simulink model "VCU_SW_1"  (R2023b)
settings: Solver=FixedStepDiscrete  StartTime=0.0  StopTime=inf  FixedStep=1e-2  RelTol=1e-3
PreLoadFcn:
  | RTWConfigurationCB('preloadfcn', bdroot);
InitFcn:
  | loadvar_ttc500
undefined symbols (not defined in the file): BrkPedalTypes, CabMovModeTypes, cFuseTempSensAcc_X, cFuseTempSensAcc_Y, cFuseTempSensVal_X, cFuseTempSensVal_Y, cTMSTempSensVal_X, cTMSTempSensVal_Y, cTransferCaseSpeedRatio, diag_state, DoorsPositionTypes, dP_filter_Y, DriverOccClassSystemTypes, ErrorValueTypes, fatal_error_callback, IO_ADC_NO_RANGE, LadderStatusTypes, pAnalogCabRotSensAcc, pAnalogCabRotSensMaxVolt, pAnalogCabRotSensMinVolt, pAnalogCabRotSensRange, pAnalogCabRotSensZeroVolt, pBrkActivePress, pCabTiltSensAcc, pCabTiltSensMaxCur, pCabTiltSensMinCur, pDistanceCorrection, pECANManual_BPNEnable, pECANManual_BPNEnabler_Flag, pFilterSensAccRes, pHDirMaxDiffFrq, pHDirSensHighLvl, pHDirSensLowLvl, pMainGearRatio, pMaxFilterSensRes, pMaxFirstPedalSensValue, pMaxFuseTempSensRes, pMaxPressLoss, pMaxPressSensCurrent, pMaxPressValue, pMaxPressValueHydMotAndPump, pMaxPressValueParkDrain, pMaxSecondPedalSensValue, pMaxTempSensVoltage, pMaxTempValue, pMaxTMSTempSensRes, pMinFilterSensRes, pMinFirstPedalSensValue, pMinFuseTempSensRes, pMinPressLoss, pMinPressSensCurrent, pMinPressValue, pMinSecondPedalSensValue, pMinTempSensVoltage, pMinTempValue, pMinTMSTempSensRes, pMotorRingTeethNum, pPedalSensAccuracyPct, pPedalSensAccuracyVolt, pPressLossTreshhold ... (+20)
libraries: TTlibrary x270, canmsglib x127, simulink x88
(part 2 of 19)

== system VCU_SW_1/ServerFcn/convDiagDataForTest ==
  convDiagDataForTest : TriggerPort  TriggerType=function-call  IsSimulinkFunction=on  FunctionName=convDiagDataForTest  VariantControl=(inherit)
  MATLAB Function : MATLAB Function  TreatAsAtomicUnit=on
  rawValue : ArgIn  DisableCoverage=on  OutDataTypeStr=uint16  ArgumentName=rawValue
  finalValue : ArgOut  DisableCoverage=on  OutDataTypeStr=uint8  ArgumentName=finalValue
  wires:
  MATLAB Function/1(canDiag) -> finalValue/1
  rawValue/1 -> MATLAB Function/1(hwDiag)

== system VCU_SW_1/ServerFcn/convINint1 ==
  convINint16fromUint16 : TriggerPort  TriggerType=function-call  IsSimulinkFunction=on  FunctionName=convINint16fromUint16  VariantControl=(inherit)
  MATLAB Function2 : MATLAB Function  TreatAsAtomicUnit=on
  x : ArgIn  DisableCoverage=on  OutDataTypeStr=int16  ArgumentName=x
  y : ArgOut  DisableCoverage=on  OutDataTypeStr=int16  ArgumentName=y
  wires:
  MATLAB Function2/1(y) -> y/1
  x/1 -> MATLAB Function2/1(x)

== system VCU_SW_1/ServerFcn/convINint16 ==
  convINint16 : TriggerPort  TriggerType=function-call  IsSimulinkFunction=on  FunctionName=convINint16  VariantControl=(inherit)
  MATLAB Function2 : MATLAB Function  TreatAsAtomicUnit=on
  x : ArgIn  DisableCoverage=on  OutDataTypeStr=single  ArgumentName=x
  y : ArgOut  DisableCoverage=on  OutDataTypeStr=int16  ArgumentName=y
  wires:
  MATLAB Function2/1(y) -> y/1
  x/1 -> MATLAB Function2/1(x)

== system VCU_SW_1/ServerFcn/convINuint16 ==
  convINuint16 : TriggerPort  TriggerType=function-call  IsSimulinkFunction=on  FunctionName=convINuint16  VariantControl=(inherit)
  MATLAB Function2 : MATLAB Function  TreatAsAtomicUnit=on
  x : ArgIn  DisableCoverage=on  OutDataTypeStr=single  ArgumentName=x
  y : ArgOut  DisableCoverage=on  OutDataTypeStr=uint16  ArgumentName=y
  wires:
  MATLAB Function2/1(y) -> y/1
  x/1 -> MATLAB Function2/1(x)

== system VCU_SW_1/ServerFcn/convPWDData ==
  convPWDData : TriggerPort  TriggerType=function-call  IsSimulinkFunction=on  FunctionName=convPWDData  VariantControl=(inherit)
  MATLAB Function : MATLAB Function  TreatAsAtomicUnit=on
  rawValue : ArgIn  DisableCoverage=on  OutDataTypeStr=uint32  ArgumentName=rawValue
  errorSts : ArgIn  Port=2  OutDataTypeStr=uint16  ArgumentName=errorSts
  finalValue : ArgOut  DisableCoverage=on  OutDataTypeStr=uint16  ArgumentName=finalValue
  wires:
  errorSts/1 -> MATLAB Function/2(errorSts)
  rawValue/1 -> MATLAB Function/1(inpValue)
  MATLAB Function/1(outValue) -> finalValue/1

== system VCU_SW_1/ServerFcn/convPWDDiagDataToEnum ==
  convPWDDiagDataToEnum : TriggerPort  TriggerType=function-call  IsSimulinkFunction=on  FunctionName=convPWDDiagDataToEnum  VariantControl=(inherit)
  Ground : Ground
  Terminator : Terminator
  rawValue : ArgIn  DisableCoverage=on  OutDataTypeStr=uint16  ArgumentName=rawValue
  enumValue : ArgOut  DisableCoverage=on  OutDataTypeStr=Enum: DigitalPinStatusTypes  ArgumentName=enumValue
  wires:
  Ground/1 -> enumValue/1
  rawValue/1 -> Terminator/1

== system VCU_SW_1/ServerFcn/convPWMDiagDataToEnum ==
  convPWMDiagDataToEnum : TriggerPort  TriggerType=function-call  IsSimulinkFunction=on  FunctionName=convPWMDiagDataToEnum  VariantControl=(inherit)
  Ground : Ground
  Terminator : Terminator
  rawValue : ArgIn  DisableCoverage=on  OutDataTypeStr=uint16  ArgumentName=rawValue
  enumValue : ArgOut  DisableCoverage=on  OutDataTypeStr=Enum: DigitalPinStatusTypes  ArgumentName=enumValue
  wires:
  Ground/1 -> enumValue/1
  rawValue/1 -> Terminator/1

== system VCU_SW_1/ServerFcn/convUintPinToenumStt ==
  convUintPinToenumStt : TriggerPort  TriggerType=function-call  IsSimulinkFunction=on  FunctionName=convUintPinToenumStt  VariantControl=(inherit)
  MATLAB Function : MATLAB Function  TreatAsAtomicUnit=on
  uintValue : ArgIn  DisableCoverage=on  OutDataTypeStr=uint8  ArgumentName=uintValue
  rawValue : ArgOut  DisableCoverage=on  OutDataTypeStr=Enum: StateModeTypes  ArgumentName=rawValue
  wires:
  uintValue/1 -> MATLAB Function/1(uintValue)
  MATLAB Function/1(enum) -> rawValue/1

== system VCU_SW_1/logSignal/getDAQCmd ==
  getDAQCmd : TriggerPort  TriggerType=function-call  IsSimulinkFunction=on  FunctionName=getDAQCmd  FunctionVisibility=scoped  VariantControl=(inherit)
  Constant : Constant  Value=uint8(1)
  Constant1 : Constant  Value=uint8(0)
  Constant2 : Constant  Value=uint8(0)
  Constant3 : Constant  Value=uint8(3)
  Terminator{,1..4} (5 alike) : Terminator
  daq_cmd_unpack : canmsglib/CAN Unpack  MsgList=(none)  MsgName=DAQ_CMD  MsgIDType=Extended (29-bit identifier)  MsgIdentifier=419364344  MsgLength=8  SignalInfo={ 'daq_cmd_ena', '0', '8', 'LE', 'unsigned', 'Standard', '0', '1', '0', '0', '255'; 'daq_cmd_page_list', '24', '8', 'LE', 'unsigned', 'Standard', '0', '1', '0', '0', '255'; 'daq_cmd_page_mode', '8', '8', 'LE', 'unsigned', 'Standard', '0', '1', '0', '0', '255'; 'daq_cmd_page_num', '16', '8', 'LE', 'unsigned', 'Standard', '0', '1', '0', '0', '255' }  IDPort=off  TimestampPort=off  ErrorPort=off  RemotePort=off  LengthPort=off  StatusPort=off  ApplyMinMax=off
  read_daq_cmd_msg : TTlibrary/CAN/read_message_name  channel=IO_CAN_CHANNEL_6  id_format=IO_CAN_EXT_FRAME  get_msg_info=off  message_names=there is no CAN Unpack blocks  message_info=|  id=419364344  ac_mask=536870911  retranslation=off  io_error=on  sample_time=-1
      | Message Name: DAQ_CMD
      |  Message ID Type: Standard (11-bit identifier)
      |  Message ID: 2
      settings: SourceProductName=TT control 500 series
  daqEna : ArgOut  OutDataTypeStr=uint8  ArgumentName=daqEna
  daqPage : ArgOut  Port=2  OutDataTypeStr=uint8  ArgumentName=daqPage
  daqList : ArgOut  Port=3  OutDataTypeStr=uint8  ArgumentName=daqList
  daqMode : ArgOut  Port=4  OutDataTypeStr=uint8  ArgumentName=daqMode
  wires:
  read_daq_cmd_msg/2 -> Terminator/1  "handler_err_419364344"
  read_daq_cmd_msg/1 -> daq_cmd_unpack/1  "msg_419364344"
  daq_cmd_unpack/1 -> Terminator1/1
  daq_cmd_unpack/2 -> Terminator2/1
  daq_cmd_unpack/3 -> Terminator3/1
  daq_cmd_unpack/4 -> Terminator4/1
  Constant/1 -> daqEna/1
  Constant1/1 -> daqMode/1
  Constant2/1 -> daqList/1
  Constant3/1 -> daqPage/1

== system VCU_SW_1/logSignal/getListData ==
  getListData : TriggerPort  TriggerType=function-call  IsSimulinkFunction=on  FunctionName=getListData  FunctionVisibility=scoped  VariantControl=(inherit)
  Simulink Function : Subsystem  TreatAsAtomicUnit=on
  Simulink Function1 : Subsystem  TreatAsAtomicUnit=on
  listData_mf : MATLAB Function  TreatAsAtomicUnit=on
  pageHighvoltageAppData : Subsystem  TreatAsAtomicUnit=on
  pageInputFcns : Subsystem  Commented=on  TreatAsAtomicUnit=on
  pageOutputRawData : Subsystem  TreatAsAtomicUnit=on
  pageRawInput : Subsystem  TreatAsAtomicUnit=on
  page : ArgIn  DisableCoverage=on  OutDataTypeStr=uint8  ArgumentName=page
  list : ArgIn  Port=2  OutDataTypeStr=uint8  ArgumentName=list
  data : ArgOut  DisableCoverage=on  OutDataTypeStr=uint8  PortDimensions=[1,7]  ArgumentName=data
  len : ArgOut  Port=2  OutDataTypeStr=uint8  ArgumentName=len
  wires:
  listData_mf/1(data) -> data/1
  listData_mf/2(len) -> len/1
  page/1 -> listData_mf/1(page)
  list/1 -> listData_mf/2(list)

== system VCU_SW_1/logSignal/getListNum ==
  getListNum : TriggerPort  TriggerType=function-call  IsSimulinkFunction=on  FunctionName=getListNum  FunctionVisibility=scoped  VariantControl=(inherit)
  MATLAB Function : MATLAB Function  TreatAsAtomicUnit=on
  page : ArgIn  DisableCoverage=on  OutDataTypeStr=uint8  ArgumentName=page
  num : ArgOut  DisableCoverage=on  OutDataTypeStr=uint8  ArgumentName=num
  wires:
  page/1 -> MATLAB Function/1(pageNum)
  MATLAB Function/1(numList) -> num/1

== system VCU_SW_1/logSignal/transmitDAQMsg ==
  transmitDAQMsg : TriggerPort  TriggerType=function-call  IsSimulinkFunction=on  FunctionName=transmitDAQMsg  FunctionVisibility=scoped  VariantControl=(inherit)
  daqPack : canmsglib/CAN Pack  MsgList=(none)  MsgName=daqPack  MsgIDType=Extended (29-bit identifier)  MsgIdentifier=419364606  MsgLength=8  Remote=off  ApplyMinMax=off  BusOutput=on  SignalInfo={}
      settings: DataFormat=raw data
  transmit_daq : TTlibrary/CAN/transmit_message_name  channel=IO_CAN_CHANNEL_6  id_format=IO_CAN_EXT_FRAME  retranslation=off  io_error=off  sample_time=-1
      settings: SourceProductName=TT control 500 series
  buffer : ArgIn  DisableCoverage=on  OutDataTypeStr=uint8  PortDimensions=[1,8]  ArgumentName=buffer
  wires:
  buffer/1 -> daqPack/1
  daqPack/1 -> transmit_daq/1

== system VCU_SW_1/EEPROM Layer/calculate trip distance/EEPROM read ==
  In1 : Inport
  function : TriggerPort  TriggerType=function-call  VariantControl=Variant
  Data Store Read1 : DataStoreRead  DataStoreName=EEPROMData  DataStoreElements=EEPROMData.savedDistM#EEPROMData.savedDistKM#EEPROMData.savedDistKKM  IndexOptions=Index vector (dialog)  Indices=1  OutputSizes=1
  Data Store Write1 : DataStoreWrite  DataStoreName=EEPROMData  DataStoreElements=EEPROMData.updatedDistM#EEPROMData.updatedDistKM#EEPROMData.updatedDistKKM  IndexOptions=Index vector (dialog)  Indices=1  OutputSizes=1
  Data Store Write2 : DataStoreWrite  DataStoreName=EEPROMData  DataStoreElements=EEPROMData.totalDistM  IndexOptions=Index vector (dialog)  Indices=1  OutputSizes=1
  Display : Display
  calcTotalDist : MATLAB Function  TreatAsAtomicUnit=on
  wires:
  calcTotalDist/4(updDistTotal) -> Display/1, Data Store Write2/1
  calcTotalDist/2(updDistKM) -> Data Store Write1/2
  Data Store Read1/1 -> calcTotalDist/2(savedDistM)
  calcTotalDist/1(updDistM) -> Data Store Write1/1
  In1/1 -> calcTotalDist/1(tripDist)
  Data Store Read1/2 -> calcTotalDist/3(savedDistKM)
  Data Store Read1/3 -> calcTotalDist/4(savedDistKKM)
  calcTotalDist/3(updDistKKM) -> Data Store Write1/3

== system VCU_SW_1/EEPROM Layer/calculate trip distance/EEPROM read1 ==
  In1 : Inport
  function : TriggerPort  TriggerType=function-call  VariantControl=Variant
  Data Store Read1 : DataStoreRead  DataStoreName=EEPROMData  DataStoreElements=EEPROMData.savedDistM_Trip#EEPROMData.savedDistKM_Trip#EEPROMData.savedDistKKM_Trip  IndexOptions=Index vector (dialog)  Indices=1  OutputSizes=1
  Data Store Write1 : DataStoreWrite  DataStoreName=EEPROMData  DataStoreElements=EEPROMData.updatedDistM_Trip#EEPROMData.updatedDistKM_Trip#EEPROMData.updatedDistKKM_Trip  IndexOptions=Index vector (dialog)  Indices=1  OutputSizes=1
  Data Store Write2 : DataStoreWrite  DataStoreName=EEPROMData  DataStoreElements=EEPROMData.totalDistM_Trip  IndexOptions=Index vector (dialog)  Indices=1  OutputSizes=1
  Display : Display
  calcTotalDist : MATLAB Function  TreatAsAtomicUnit=on
  wires:
  calcTotalDist/3(updDistKKM) -> Data Store Write1/3
  Data Store Read1/3 -> calcTotalDist/4(savedDistKKM)
  Data Store Read1/2 -> calcTotalDist/3(savedDistKM)
  In1/1 -> calcTotalDist/1(tripDist)
  calcTotalDist/1(updDistM) -> Data Store Write1/1
  Data Store Read1/1 -> calcTotalDist/2(savedDistM)
  calcTotalDist/2(updDistKM) -> Data Store Write1/2
  calcTotalDist/4(updDistTotal) -> Data Store Write2/1, Display/1

== system VCU_SW_1/InputData/InputData/AnalogInputs ==
  AcceleratorPedalSens1 : TTlibrary/ADC/adcGetValue  Commented=on  adc_channel=IO_ADC_58  types=IO_ADC_RATIOMETRIC  range=IO_ADC_NO_RANGE:  pupd=IO_ADC_PU_10K  sensor_supply=IO_SENSOR_SUPPLY_1  safety_conf=off  adc_val_lower=4  adc_val_upper=4  redundant_channel=IO_ADC_08  io_error=on  sample_time=-1
      settings: SourceProductName=TT control 500 series
  AcceleratorPedalSens3 : TTlibrary/ADC/adcGetValue  Commented=on  adc_channel=IO_ADC_02  types=IO_ADC_RATIOMETRIC  range=IO_ADC_NO_RANGE  pupd=IO_ADC_NO_PULL  sensor_supply=IO_SENSOR_SUPPLY_1  safety_conf=off  adc_val_lower=4  adc_val_upper=4  redundant_channel=IO_ADC_08  io_error=on  sample_time=-1
      settings: SourceProductName=TT control 500 series
  Data Store Write1 : DataStoreWrite  Commented=on  DataStoreName=OutputNetworkData  DataStoreElements=OutputNetworkData.Pin101_Pin104_FB.Pin1_feedback  IndexOptions=Index vector (dialog)  Indices=1  OutputSizes=1
  Data Store Write7 : DataStoreWrite  Commented=on  DataStoreName=OutputNetworkData  DataStoreElements=OutputNetworkData.Pin101_Pin104_FB.Pin0_feedback  IndexOptions=Index vector (dialog)  Indices=1  OutputSizes=1
  Function Caller1 : FunctionCaller  Commented=on  FunctionPrototype=finalValue = convAIVoltageData(rawValue,errorSts)  InputArgumentSpecifications=<Enter example>  OutputArgumentSpecifications=<Enter example>
  Function Caller3 : FunctionCaller  Commented=on  FunctionPrototype=finalValue = convAIVoltageData(rawValue,errorSts)  InputArgumentSpecifications=<Enter example>  OutputArgumentSpecifications=<Enter example>
  Terminator1 : Terminator  Commented=on
  Terminator3 : Terminator  Commented=on
  wires:
  AcceleratorPedalSens3/3 -> Function Caller3/2  "adc_104_error"
  AcceleratorPedalSens3/2 -> Terminator3/1  "adc_104_update"
  Function Caller3/1 -> Data Store Write7/1
  AcceleratorPedalSens3/1 -> Function Caller3/1  "adc_104_value"
  AcceleratorPedalSens1/1 -> Function Caller1/1  "adc_194_value"
  AcceleratorPedalSens1/2 -> Terminator1/1  "adc_194_update"
  AcceleratorPedalSens1/3 -> Function Caller1/2  "adc_194_error"
  Function Caller1/1 -> Data Store Write1/1

== system VCU_SW_1/InputData/InputData/DigitalInputs ==
  note: по доке PD_2_5
  note: по доке PD_2_5
  Data Store Write1 : DataStoreWrite  Commented=on  DataStoreName=OutputNetworkData  DataStoreElements=OutputNetworkData.Pin101_Pin104_FB.Pin0_feedback  IndexOptions=Index vector (dialog)  Indices=1  OutputSizes=1
  Data Store Write13 : DataStoreWrite  DataStoreName=OutputNetworkData  DataStoreElements=OutputNetworkData.Pin101_Pin104_FB.Pin0_feedback  IndexOptions=Index vector (dialog)  Indices=1  OutputSizes=1
  Data Type Conversion : DataTypeConversion  OutDataTypeStr=uint16  SaturateOnIntegerOverflow=off  RndMeth=Floor
  Data Type Conversion1 : DataTypeConversion  Commented=on  OutDataTypeStr=uint16  SaturateOnIntegerOverflow=off  RndMeth=Floor
  EngineAirFilterClogSens : TTlibrary/DIO/getDigitalInputValue  di_channel=IO_DI_50  pupd=IO_DI_PU_10K  limits=off  low_thresh1=0  low_thresh2=2500  high_thresh1=2500  high_thresh2=32000  io_error=on  sample_time=-1
      settings: SourceProductName=TT control 500 series
  ExtrRightCabinePosSens : TTlibrary/DIO/getDigitalInputValue  Commented=on  di_channel=IO_DI_94  pupd=IO_DI_PD_10K  limits=off  low_thresh1=0  low_thresh2=2500  high_thresh1=2500  high_thresh2=32000  io_error=on  sample_time=-1
      settings: SourceProductName=TT control 500 series
  Function Caller13 : FunctionCaller  FunctionPrototype=enumValue = convDIOSttToEnum(rawValue,errorSts)  InputArgumentSpecifications=<Enter example>  OutputArgumentSpecifications=<Enter example>
  Function Caller17 : FunctionCaller  Commented=on  FunctionPrototype=enumValue = convDIOSttToEnum(rawValue,errorSts)  InputArgumentSpecifications=<Enter example>  OutputArgumentSpecifications=<Enter example>
  wires:
  Data Type Conversion/1 -> Data Store Write13/1
  EngineAirFilterClogSens/2 -> Function Caller13/2  "di_104_error"
  Function Caller13/1 -> Data Type Conversion/1
  EngineAirFilterClogSens/1 -> Function Caller13/1  "di_104_value"
  ExtrRightCabinePosSens/1 -> Function Caller17/1  "di_194_value"
  ExtrRightCabinePosSens/2 -> Function Caller17/2  "di_194_error"
  Function Caller17/1 -> Data Type Conversion1/1
  Data Type Conversion1/1 -> Data Store Write1/1

== system VCU_SW_1/InputLayer/InputInterfaces/AnalogInput ==
  1000msec : simulink/Ports & Subsystems/Function-Call Generator  sample_time=1  numberOfIterations=1  DisallowWideOutput=off
  100msec : simulink/Ports & Subsystems/Function-Call Generator  sample_time=0.1  numberOfIterations=1  DisallowWideOutput=off
  10msec : simulink/Ports & Subsystems/Function-Call Generator  sample_time=0.01  numberOfIterations=1  DisallowWideOutput=off
  AIProc1000msec : Subsystem  TreatAsAtomicUnit=on
      settings: RTWSystemCode=Nonreusable function
  AIProc100msec : Subsystem  TreatAsAtomicUnit=on
      settings: RTWSystemCode=Nonreusable function
  AIProc10msec : Subsystem  TreatAsAtomicUnit=on
      settings: RTWSystemCode=Nonreusable function
  Function-Call Split : FunctionCallSplit  NumOutputPorts=2  OutputPortLayout=default
  Function-Call Split1 : FunctionCallSplit  NumOutputPorts=2  OutputPortLayout=default
  Function-Call Split2 : FunctionCallSplit  NumOutputPorts=2  OutputPortLayout=default
  GetAI1000msec : Subsystem  TreatAsAtomicUnit=on
      settings: RTWSystemCode=Nonreusable function
  GetAI100msec : Subsystem  TreatAsAtomicUnit=on
      settings: RTWSystemCode=Nonreusable function
  GetAI10msec : Subsystem  TreatAsAtomicUnit=on
      settings: RTWSystemCode=Nonreusable function
  wires:
  1000msec/1 -> Function-Call Split2/1
  100msec/1 -> Function-Call Split1/1
  10msec/1 -> Function-Call Split/1
  Function-Call Split/2 -> GetAI10msec/Trigger
  Function-Call Split/1 -> AIProc10msec/Trigger
  Function-Call Split1/1 -> AIProc100msec/Trigger
  Function-Call Split1/2 -> GetAI100msec/Trigger
  Function-Call Split2/1 -> AIProc1000msec/Trigger
  Function-Call Split2/2 -> GetAI1000msec/Trigger

== system VCU_SW_1/InputLayer/InputInterfaces/DigitalInput ==
  note: Для форвардера
  note: Вместо вызывальщика завести обратную свзяь по питанию этого датчика - когда оно появилось - ждем секунду и начинаем обработку, до того момента шлем значения, как будто кабина в нулевом положении (по моему это два нуля на датчиках).
  note: Убрать внутренний вызывальщик, передачу данных из подсистемы getDI сделать прямым пробросом, внутри убрать функции на считывания и записи
  1000msec : simulink/Ports & Subsystems/Function-Call Generator  sample_time=1  numberOfIterations=1  DisallowWideOutput=off
  100msec : simulink/Ports & Subsystems/Function-Call Generator  sample_time=0.1  numberOfIterations=1  DisallowWideOutput=off
  10msec : simulink/Ports & Subsystems/Function-Call Generator  sample_time=0.01  numberOfIterations=1  DisallowWideOutput=off
  Function-Call Split : FunctionCallSplit  NumOutputPorts=2  OutputPortLayout=default
  Function-Call Split1 : FunctionCallSplit  NumOutputPorts=2  OutputPortLayout=default
  Function-Call Subsystem : Subsystem  TreatAsAtomicUnit=on
  Function-Call Subsystem1 : Subsystem  TreatAsAtomicUnit=on
  Function-Call Subsystem2 : Subsystem  TreatAsAtomicUnit=on
  GetDI1000msec : Subsystem  TreatAsAtomicUnit=on
      settings: RTWSystemCode=Nonreusable function
  GetDI100msec : Subsystem  TreatAsAtomicUnit=on
      settings: RTWSystemCode=Nonreusable function
  GetDI10msec : Subsystem  TreatAsAtomicUnit=on
      settings: RTWSystemCode=Nonreusable function
  wires:
  10msec/1 -> Function-Call Split/1
  1000msec/1 -> GetDI1000msec/Trigger
  100msec/1 -> Function-Call Split1/1
  Function-Call Split/2 -> GetDI10msec/Trigger
  Function-Call Split1/2 -> GetDI100msec/Trigger
  Function-Call Split/1 -> Function-Call Subsystem/Trigger
  Function-Call Split1/1 -> Function-Call Subsystem1/Trigger

== system VCU_SW_1/InputLayer/InputInterfaces/PWDInput ==
  1000msec : simulink/Ports & Subsystems/Function-Call Generator  sample_time=1  numberOfIterations=1  DisallowWideOutput=off
  100msec : simulink/Ports & Subsystems/Function-Call Generator  sample_time=0.1  numberOfIterations=1  DisallowWideOutput=off
  10msec : simulink/Ports & Subsystems/Function-Call Generator  sample_time=0.01  numberOfIterations=1  DisallowWideOutput=off
  Function-Call Split1 : FunctionCallSplit  NumOutputPorts=2  OutputPortLayout=default
  GetPWD1000msec : Subsystem  TreatAsAtomicUnit=on
      settings: RTWSystemCode=Nonreusable function
  GetPWD100msec : Subsystem  TreatAsAtomicUnit=on
      settings: RTWSystemCode=Nonreusable function
  GetPWD10msec : Subsystem  TreatAsAtomicUnit=on
      settings: RTWSystemCode=Nonreusable function
  PWDProc100msec : Subsystem  TreatAsAtomicUnit=on
      settings: RTWSystemCode=Nonreusable function
  wires:
  100msec/1 -> Function-Call Split1/1
  Function-Call Split1/1 -> PWDProc100msec/Trigger
  Function-Call Split1/2 -> GetPWD100msec/Trigger
  10msec/1 -> GetPWD10msec/Trigger
  1000msec/1 -> GetPWD1000msec/Trigger

== system VCU_SW_1/InputLayer/InputInterfaces/PWMCurrentInput ==
  1000msec : simulink/Ports & Subsystems/Function-Call Generator  sample_time=1  numberOfIterations=1  DisallowWideOutput=off
  100msec : simulink/Ports & Subsystems/Function-Call Generator  sample_time=0.1  numberOfIterations=1  DisallowWideOutput=off
  10msec : simulink/Ports & Subsystems/Function-Call Generator  sample_time=0.01  numberOfIterations=1  DisallowWideOutput=off
  Function-Call Split : FunctionCallSplit  NumOutputPorts=2  OutputPortLayout=default
  GetPWMCur1000msec : Subsystem  TreatAsAtomicUnit=on
      settings: RTWSystemCode=Nonreusable function
  GetPWMCur100msec : Subsystem  TreatAsAtomicUnit=on
      settings: RTWSystemCode=Nonreusable function
  GetPWMCur10msec : Subsystem  TreatAsAtomicUnit=on
      settings: RTWSystemCode=Nonreusable function
  PWMCur10msecProc : Subsystem  TreatAsAtomicUnit=on
      settings: RTWSystemCode=Nonreusable function
  wires:
  Function-Call Split/1 -> PWMCur10msecProc/Trigger
  Function-Call Split/2 -> GetPWMCur10msec/Trigger
  10msec/1 -> Function-Call Split/1
  100msec/1 -> GetPWMCur100msec/Trigger
  1000msec/1 -> GetPWMCur1000msec/Trigger

== system VCU_SW_1/InputLayer/InputNetwork/InputCCAN ==
  note: костыльно сделано что водила есть всегда
  note: Удалить если не несет смысловой нагрузки
  note: Нам все подряд сообщения не нужны, но в целом можно оставить
  1000msec : simulink/Ports & Subsystems/Function-Call Generator  sample_time=1  numberOfIterations=1  DisallowWideOutput=off
  100msec : simulink/Ports & Subsystems/Function-Call Generator  sample_time=0.1  numberOfIterations=1  DisallowWideOutput=off
  10msec : simulink/Ports & Subsystems/Function-Call Generator  Commented=on  sample_time=0.01  numberOfIterations=1  DisallowWideOutput=off
  200msec : simulink/Ports & Subsystems/Function-Call Generator  Commented=on  sample_time=0.2  numberOfIterations=1  DisallowWideOutput=off
  500msec : simulink/Ports & Subsystems/Function-Call Generator  sample_time=0.5  numberOfIterations=1  DisallowWideOutput=off
  CCAN100msecProc1 : Subsystem  TreatAsAtomicUnit=on
      settings: RTWSystemCode=Nonreusable function
  "CCAN10msecProc " : Subsystem  Commented=on  TreatAsAtomicUnit=on
      settings: RTWSystemCode=Nonreusable function
  Function-Call Split : FunctionCallSplit  Commented=on  NumOutputPorts=2  OutputPortLayout=default
  Function-Call Split1 : FunctionCallSplit  NumOutputPorts=2  OutputPortLayout=default
  GetCCAN1000msec : Subsystem  TreatAsAtomicUnit=on
      settings: RTWSystemCode=Nonreusable function
  GetCCAN100msec : Subsystem  TreatAsAtomicUnit=on
      settings: RTWSystemCode=Nonreusable function
  GetCCAN10msec : Subsystem  Commented=on  TreatAsAtomicUnit=on
      settings: RTWSystemCode=Nonreusable function
  GetCCAN200msec : Subsystem  Commented=on  TreatAsAtomicUnit=on
      settings: RTWSystemCode=Nonreusable function
  GetCCAN500msec : Subsystem  TreatAsAtomicUnit=on
      settings: RTWSystemCode=Nonreusable function
  wires:
  Function-Call Split1/2 -> GetCCAN100msec/Trigger
  Function-Call Split1/1 -> CCAN100msecProc1/Trigger
  Function-Call Split/2 -> GetCCAN10msec/Trigger
  Function-Call Split/1 -> "CCAN10msecProc "/Trigger
  100msec/1 -> Function-Call Split1/1
  500msec/1 -> GetCCAN500msec/Trigger
  200msec/1 -> GetCCAN200msec/Trigger
  10msec/1 -> Function-Call Split/1
  1000msec/1 -> GetCCAN1000msec/Trigger

== system VCU_SW_1/InputLayer/InputNetwork/InputDiagCAN ==
  10msec : simulink/Ports & Subsystems/Function-Call Generator  Commented=on  sample_time=0.01  numberOfIterations=1  DisallowWideOutput=off
  10msec1 : simulink/Ports & Subsystems/Function-Call Generator  sample_time=0.01  numberOfIterations=1  DisallowWideOutput=off
  GetDiagCAN10msec : Subsystem  Commented=on  TreatAsAtomicUnit=on
      settings: RTWSystemCode=Nonreusable function
  GetDiagCAN10msec1 : Subsystem  TreatAsAtomicUnit=on
      settings: RTWSystemCode=Nonreusable function
  wires:
  10msec/1 -> GetDiagCAN10msec/Trigger
  10msec1/1 -> GetDiagCAN10msec1/Trigger

== system VCU_SW_1/InputLayer/InputNetwork/InputEngCAN ==
  note: EngCAN
      |
      | In
      |
      | ECU_EEC1 00 +
      | ECU_EEC2 00 +
      | ECU_EEC3 00 +
      | ECU_ET1 00 +
      | ECU_ET2 00 +
      | ECU_LFE1 00 +
      | ECU_SHUTDN 00 +
      | ECU_TPCM 00, ECU_TPDT 00 (так блин нафик, это вот тут вот мультипакет, он не сделан)
      | ECU_VEP1 00 +
      |
      | Отдельный вопрос - что из этого необходимо
  note: EngCAN
      |
      | Out
      |
      | VCU_ECU_TSC1 FA
  note: Мультипакет закомментирован
  1000msec : simulink/Ports & Subsystems/Function-Call Generator  sample_time=1  numberOfIterations=1  DisallowWideOutput=off
  100msec : simulink/Ports & Subsystems/Function-Call Generator  sample_time=0.1  numberOfIterations=1  DisallowWideOutput=off
  250msec : simulink/Ports & Subsystems/Function-Call Generator  sample_time=0.25  numberOfIterations=1  DisallowWideOutput=off
  500msec : simulink/Ports & Subsystems/Function-Call Generator  sample_time=0.5  numberOfIterations=1  DisallowWideOutput=off
  50msec : simulink/Ports & Subsystems/Function-Call Generator  sample_time=0.05  numberOfIterations=1  DisallowWideOutput=off
  GetEngCAN1000msec : Subsystem  TreatAsAtomicUnit=on
      settings: RTWSystemCode=Nonreusable function
  GetEngCAN100msec : Subsystem  TreatAsAtomicUnit=on
      settings: RTWSystemCode=Nonreusable function
  GetEngCAN250msec : Subsystem  TreatAsAtomicUnit=on
      settings: RTWSystemCode=Nonreusable function
  GetEngCAN500msec : Subsystem  TreatAsAtomicUnit=on
      settings: RTWSystemCode=Nonreusable function
  GetEngCAN50msec : Subsystem  TreatAsAtomicUnit=on
      settings: RTWSystemCode=Nonreusable function
  wires:
  500msec/1 -> GetEngCAN500msec/Trigger
  250msec/1 -> GetEngCAN250msec/Trigger
  50msec/1 -> GetEngCAN50msec/Trigger
  1000msec/1 -> GetEngCAN1000msec/Trigger
  100msec/1 -> GetEngCAN100msec/Trigger

== system VCU_SW_1/InputLayer/InputNetwork/InputHydCAN ==
  100msec : simulink/Ports & Subsystems/Function-Call Generator  sample_time=0.1  numberOfIterations=1  DisallowWideOutput=off
  GetHydCAN100msec : Subsystem  TreatAsAtomicUnit=on
      settings: RTWSystemCode=Nonreusable function
  wires:
  100msec/1 -> GetHydCAN100msec/Trigger

== system VCU_SW_1/InputLayer/InputNetwork/InputStrCAN ==
  100msec : simulink/Ports & Subsystems/Function-Call Generator  sample_time=0.1  numberOfIterations=1  DisallowWideOutput=off
  Function-Call Split : FunctionCallSplit  NumOutputPorts=2  OutputPortLayout=default
  Function-Call Subsystem : Subsystem  TreatAsAtomicUnit=on
  GetStrCAN100msec : Subsystem  TreatAsAtomicUnit=on
      settings: RTWSystemCode=Nonreusable function
  wires:
  100msec/1 -> Function-Call Split/1
  Function-Call Split/2 -> GetStrCAN100msec/Trigger
  Function-Call Split/1 -> Function-Call Subsystem/Trigger

== system VCU_SW_1/InputLayer/InputNetwork/InputxCraneCAN ==
  note: только PUMPS
  100msec : simulink/Ports & Subsystems/Function-Call Generator  sample_time=0.1  numberOfIterations=1  DisallowWideOutput=off
  GetxCraneCAN100msec : Subsystem  TreatAsAtomicUnit=on
      settings: RTWSystemCode=Nonreusable function
  wires:
  100msec/1 -> GetxCraneCAN100msec/Trigger

== system VCU_SW_1/InputLayer/Manual/GetManual ==
  function : TriggerPort  TriggerType=function-call  VariantControl=Variant
  Cabin angles + cabin control : Subsystem
  DO : Subsystem
  EEC2 : Subsystem
  PWM : Subsystem
  Params : Subsystem
  TSC1 : Subsystem
  VLVCMD_HYD : Subsystem
  VLVCMD_STR : Subsystem

== system VCU_SW_1/OutputLayer/OutputInterfaces/DigitalOutput1 ==
  note: Привод вентилятора 195 пин
  1000msec : simulink/Ports & Subsystems/Function-Call Generator  sample_time=1  numberOfIterations=1  DisallowWideOutput=off
  100msec : simulink/Ports & Subsystems/Function-Call Generator  sample_time=0.1  numberOfIterations=1  DisallowWideOutput=off
  10msec : simulink/Ports & Subsystems/Function-Call Generator  sample_time=0.01  numberOfIterations=1  DisallowWideOutput=off
  SetDO1000msec : Subsystem  TreatAsAtomicUnit=on
      settings: RTWSystemCode=Nonreusable function
  SetDO100msec : Subsystem  TreatAsAtomicUnit=on
      settings: RTWSystemCode=Nonreusable function
  SetDO10msec : Subsystem  TreatAsAtomicUnit=on
      settings: RTWSystemCode=Nonreusable function
  wires:
  100msec/1 -> SetDO100msec/Trigger
  1000msec/1 -> SetDO1000msec/Trigger
  10msec/1 -> SetDO10msec/Trigger

== system VCU_SW_1/OutputLayer/OutputInterfaces/PWMOutput ==
  1000msec : simulink/Ports & Subsystems/Function-Call Generator  sample_time=1  numberOfIterations=1  DisallowWideOutput=off
  10msec : simulink/Ports & Subsystems/Function-Call Generator  sample_time=0.01  numberOfIterations=1  DisallowWideOutput=off
  SetPWM1000msec : Subsystem  TreatAsAtomicUnit=on
      settings: RTWSystemCode=Nonreusable function
  SetPWM10msec : Subsystem  TreatAsAtomicUnit=on
      settings: RTWSystemCode=Nonreusable function
  wires:
  1000msec/1 -> SetPWM1000msec/Trigger
  10msec/1 -> SetPWM10msec/Trigger

== system VCU_SW_1/OutputLayer/OutputInterfaces/exDigitalOutput ==
  note: Привод вентилятора 195 пин
  1000msec : simulink/Ports & Subsystems/Function-Call Generator  sample_time=1  numberOfIterations=1  DisallowWideOutput=off
  100msec : simulink/Ports & Subsystems/Function-Call Generator  sample_time=0.1  numberOfIterations=1  DisallowWideOutput=off
  10msec : simulink/Ports & Subsystems/Function-Call Generator  sample_time=0.01  numberOfIterations=1  DisallowWideOutput=off
  SetDO1000msec : Subsystem  TreatAsAtomicUnit=on
      settings: RTWSystemCode=Nonreusable function
  SetDO100msec : Subsystem  TreatAsAtomicUnit=on
      settings: RTWSystemCode=Nonreusable function
  SetDO10msec : Subsystem  TreatAsAtomicUnit=on
      settings: RTWSystemCode=Nonreusable function
  wires:
  100msec/1 -> SetDO100msec/Trigger
  1000msec/1 -> SetDO1000msec/Trigger
  10msec/1 -> SetDO10msec/Trigger

== system VCU_SW_1/OutputLayer/OutputNetwork/OutputCCAN ==
  1000msec : simulink/Ports & Subsystems/Function-Call Generator  sample_time=1  numberOfIterations=1  DisallowWideOutput=off
  100msec : simulink/Ports & Subsystems/Function-Call Generator  sample_time=0.1  numberOfIterations=1  DisallowWideOutput=off
  10msec : simulink/Ports & Subsystems/Function-Call Generator  sample_time=0.01  numberOfIterations=1  DisallowWideOutput=off
  500msec : simulink/Ports & Subsystems/Function-Call Generator  sample_time=0.5  numberOfIterations=1  DisallowWideOutput=off
  50msec : simulink/Ports & Subsystems/Function-Call Generator  sample_time=0.05  numberOfIterations=1  DisallowWideOutput=off
  SetCCAN1000msec : Subsystem  TreatAsAtomicUnit=on
      settings: RTWSystemCode=Nonreusable function
  SetCCAN100msec : Subsystem  TreatAsAtomicUnit=on
      settings: RTWSystemCode=Nonreusable function
  SetCCAN10msec : Subsystem  TreatAsAtomicUnit=on
      settings: RTWSystemCode=Nonreusable function
  SetCCAN500msec : Subsystem  TreatAsAtomicUnit=on
      settings: RTWSystemCode=Nonreusable function
  SetCCAN50msec : Subsystem  TreatAsAtomicUnit=on
      settings: RTWSystemCode=Nonreusable function
  wires:
  10msec/1 -> SetCCAN10msec/Trigger
  50msec/1 -> SetCCAN50msec/Trigger
  1000msec/1 -> SetCCAN1000msec/Trigger
  100msec/1 -> SetCCAN100msec/Trigger
  500msec/1 -> SetCCAN500msec/Trigger

== system VCU_SW_1/OutputLayer/OutputNetwork/OutputDiagCAN + Logger ==
  100msec : simulink/Ports & Subsystems/Function-Call Generator  sample_time=0.1  numberOfIterations=1  DisallowWideOutput=off
  10msec : simulink/Ports & Subsystems/Function-Call Generator  Commented=on  sample_time=0.01  numberOfIterations=1  DisallowWideOutput=off
  10msec1 : simulink/Ports & Subsystems/Function-Call Generator  sample_time=0.01  numberOfIterations=1  DisallowWideOutput=off
  LOGGER : Subsystem  TreatAsAtomicUnit=on
      settings: RTWSystemCode=Nonreusable function
  SetDiagCAN10msec : Subsystem  Commented=on  TreatAsAtomicUnit=on
      settings: RTWSystemCode=Nonreusable function
  SetDiagCAN10msec1 : Subsystem  TreatAsAtomicUnit=on
      settings: RTWSystemCode=Nonreusable function
  exLogger : Subsystem  Commented=on  TreatAsAtomicUnit=on
      settings: RTWSystemCode=Nonreusable function
  wires:
  100msec/1 -> LOGGER/Trigger
  10msec/1 -> SetDiagCAN10msec/Trigger
  10msec1/1 -> SetDiagCAN10msec1/Trigger

== system VCU_SW_1/OutputLayer/OutputNetwork/OutputEngCAN ==
  50msec : simulink/Ports & Subsystems/Function-Call Generator  sample_time=0.05  numberOfIterations=1  DisallowWideOutput=off
  SetEngCAN50msec : Subsystem  TreatAsAtomicUnit=on
      settings: RTWSystemCode=Nonreusable function
  wires:
  50msec/1 -> SetEngCAN50msec/Trigger

== system VCU_SW_1/OutputLayer/OutputNetwork/OutputHydCAN ==
  100msec : simulink/Ports & Subsystems/Function-Call Generator  sample_time=0.1  numberOfIterations=1  DisallowWideOutput=off
  SetHydCAN100msec : Subsystem  TreatAsAtomicUnit=on
      settings: RTWSystemCode=Nonreusable function
  wires:
  100msec/1 -> SetHydCAN100msec/Trigger

== system VCU_SW_1/OutputLayer/OutputNetwork/OutputStrCAN ==
  100msec : simulink/Ports & Subsystems/Function-Call Generator  sample_time=0.01  numberOfIterations=1  DisallowWideOutput=off
  SetStrCAN100msec : Subsystem  TreatAsAtomicUnit=on
      settings: RTWSystemCode=Nonreusable function
  wires:
  100msec/1 -> SetStrCAN100msec/Trigger

== system VCU_SW_1/OutputLayer/OutputNetwork/OutputxCraneCAN ==

== system VCU_SW_1/logSignal/getListData/Simulink Function ==
  splitIntoTwoBytes : TriggerPort  TriggerType=function-call  IsSimulinkFunction=on  FunctionName=splitIntoTwoBytes  FunctionVisibility=scoped  VariantControl=(inherit)
  MATLAB Function : MATLAB Function  TreatAsAtomicUnit=on
  Mux : Mux  Inputs=2
  value : ArgIn  DisableCoverage=on  OutDataTypeStr=uint16  ArgumentName=value
  data : ArgOut  DisableCoverage=on  OutDataTypeStr=uint8  PortDimensions=[1,2]  ArgumentName=data
  wires:
  value/1 -> MATLAB Function/1(value)
  MATLAB Function/1(byte1) -> Mux/1
  MATLAB Function/2(byte2) -> Mux/2
  Mux/1 -> data/1

== system VCU_SW_1/logSignal/getListData/Simulink Function1 ==
  splitIntoFourBytes : TriggerPort  TriggerType=function-call  IsSimulinkFunction=on  FunctionName=splitIntoFourBytes  FunctionVisibility=scoped  VariantControl=(inherit)
  MATLAB Function : MATLAB Function  TreatAsAtomicUnit=on
  Mux : Mux
  value : ArgIn  DisableCoverage=on  OutDataTypeStr=uint32  ArgumentName=value
  data : ArgOut  DisableCoverage=on  OutDataTypeStr=uint8  PortDimensions=[1,4]  ArgumentName=data
  wires:
  value/1 -> MATLAB Function/1(value)
  MATLAB Function/1(byte1) -> Mux/1
  MATLAB Function/2(byte2) -> Mux/2
  MATLAB Function/3(byte3) -> Mux/3
  MATLAB Function/4(byte4) -> Mux/4
  Mux/1 -> data/1

== system VCU_SW_1/logSignal/getListData/pageHighvoltageAppData ==
  note: инвертора
  pageHighvoltageAppData : TriggerPort  TriggerType=function-call  IsSimulinkFunction=on  FunctionName=pageHighvoltageAppData  FunctionVisibility=scoped  VariantControl=(inherit)
  MATLAB Function : MATLAB Function  TreatAsAtomicUnit=on
  getListDataII1 : Subsystem  TreatAsAtomicUnit=on
  getListDataII10 : Subsystem  TreatAsAtomicUnit=on
  getListDataII11 : Subsystem  TreatAsAtomicUnit=on
  getListDataII12 : Subsystem  TreatAsAtomicUnit=on
  getListDataII2 : Subsystem  TreatAsAtomicUnit=on
  getListDataII3 : Subsystem  TreatAsAtomicUnit=on
  getListDataII4 : Subsystem  TreatAsAtomicUnit=on
  getListDataII5 : Subsystem  TreatAsAtomicUnit=on
  getListDataII6 : Subsystem  TreatAsAtomicUnit=on
  getListDataII7 : Subsystem  TreatAsAtomicUnit=on
  getListDataII8 : Subsystem  TreatAsAtomicUnit=on
  getListDataII9 : Subsystem  TreatAsAtomicUnit=on
  list : ArgIn  OutDataTypeStr=uint8  ArgumentName=list
  data : ArgOut  DisableCoverage=on  OutDataTypeStr=uint8  PortDimensions=[1,7]  ArgumentName=data
  len : ArgOut  Port=2  OutDataTypeStr=uint8  ArgumentName=len
  wires:
  MATLAB Function/2(len) -> len/1
  MATLAB Function/1(data) -> data/1
  list/1 -> MATLAB Function/1(list)

== system VCU_SW_1/logSignal/getListData/pageInputFcns ==
  pageInputFcns : TriggerPort  TriggerType=function-call  IsSimulinkFunction=on  FunctionName=pageInputFcns  FunctionVisibility=scoped  VariantControl=(inherit)
  list : ArgIn  ArgumentName=list
  data : ArgOut  DisableCoverage=on  ArgumentName=data
  wires:
  ? -> data/1

== system VCU_SW_1/logSignal/getListData/pageOutputRawData ==
  pageOutputRawData : TriggerPort  TriggerType=function-call  IsSimulinkFunction=on  FunctionName=pageOutputRawData  FunctionVisibility=scoped  VariantControl=(inherit)
  MATLAB Function : MATLAB Function  TreatAsAtomicUnit=on
  getListDataOI1 : Subsystem  TreatAsAtomicUnit=on
  getListDataOI2 : Subsystem  TreatAsAtomicUnit=on
  getListDataOI3 : Subsystem  TreatAsAtomicUnit=on
  list : ArgIn  OutDataTypeStr=uint8  ArgumentName=list
  data : ArgOut  DisableCoverage=on  OutDataTypeStr=uint8  PortDimensions=[1,7]  ArgumentName=data
  wires:
  MATLAB Function/1(data) -> data/1
  list/1 -> MATLAB Function/1(list)

== system VCU_SW_1/logSignal/getListData/pageRawInput ==
  pageRawInput : TriggerPort  TriggerType=function-call  IsSimulinkFunction=on  FunctionName=pageRawInput  FunctionVisibility=scoped  VariantControl=(inherit)
  MATLAB Function : MATLAB Function  TreatAsAtomicUnit=on
  getListDataII1 : Subsystem  TreatAsAtomicUnit=on
  getListDataII2 : Subsystem  TreatAsAtomicUnit=on
  getListDataII3 : Subsystem  TreatAsAtomicUnit=on
  getListDataII4 : Subsystem  TreatAsAtomicUnit=on
  getListDataII5 : Subsystem  TreatAsAtomicUnit=on
  getListDataII6 : Subsystem  TreatAsAtomicUnit=on
  getListDataII7 : Subsystem  TreatAsAtomicUnit=on
  getListDataII8 : Subsystem  TreatAsAtomicUnit=on
  list : ArgIn  DisableCoverage=on  OutDataTypeStr=uint8  ArgumentName=list
  data : ArgOut  DisableCoverage=on  OutDataTypeStr=uint8  PortDimensions=[1,7]  ArgumentName=data
  len : ArgOut  Port=2  OutDataTypeStr=uint8  ArgumentName=len
  wires:
  list/1 -> MATLAB Function/1(list)
  MATLAB Function/1(data) -> data/1
  MATLAB Function/2(len) -> len/1

== system VCU_SW_1/InputLayer/InputInterfaces/AnalogInput/AIProc1000msec ==
  function : TriggerPort  TriggerType=function-call  VariantControl=Variant
  Filter : Subsystem  TreatAsAtomicUnit=on
  TemperatureValues : Subsystem  TreatAsAtomicUnit=on

== system VCU_SW_1/InputLayer/InputInterfaces/AnalogInput/AIProc100msec ==
  function : TriggerPort  TriggerType=function-call  VariantControl=Variant
  GenWorkSig : Subsystem
  PressureValues : Subsystem  TreatAsAtomicUnit=on

== system VCU_SW_1/InputLayer/InputInterfaces/AnalogInput/AIProc10msec ==
  note: Тут есть ньюанс, именно из анекдота
  function : TriggerPort  TriggerType=function-call  VariantControl=Variant
  CabMovValues : Subsystem  TreatAsAtomicUnit=on
  MATLAB Function : MATLAB Function  TreatAsAtomicUnit=on
  PedalValues : Subsystem  TreatAsAtomicUnit=on
  PressureValues : Subsystem  TreatAsAtomicUnit=on
  PumpMotorDirections : Subsystem  TreatAsAtomicUnit=on
  WasherTiltPumpTrans : Subsystem  TreatAsAtomicUnit=on
  wires:
  MATLAB Function/1(fcncall()) -> CabMovValues/Trigger

== system VCU_SW_1/InputLayer/InputInterfaces/AnalogInput/GetAI1000msec ==
  function : TriggerPort  TriggerType=function-call  VariantControl=Variant
  Data Store Write1 : DataStoreWrite  DataStoreName=UDSStruct  DataStoreElements=UDSStruct.pin_filterClogSens  IndexOptions=Index vector (dialog)  Indices=1  OutputSizes=1
  Data Store Write12 : DataStoreWrite  DataStoreName=InputInterfaceData  DataStoreElements=InputInterfaceData.AI.hydMotTempSens  IndexOptions=Index vector (dialog)  Indices=1  OutputSizes=1
  Data Store Write2 : DataStoreWrite  DataStoreName=UDSStruct  DataStoreElements=UDSStruct.pin_hydMotTempSens  IndexOptions=Index vector (dialog)  Indices=1  OutputSizes=1
  Data Store Write23 : DataStoreWrite  DataStoreName=InputInterfaceData  DataStoreElements=InputInterfaceData.AI.transPumpTempSens  IndexOptions=Index vector (dialog)  Indices=1  OutputSizes=1
  Data Store Write26 : DataStoreWrite  DataStoreName=LogInputInterfaceData  DataStoreElements=LogInputInterfaceData.AI_1_Log.log_filterClogSens  IndexOptions=Index vector (dialog)  Indices=1  OutputSizes=1
  Data Store Write28 : DataStoreWrite  DataStoreName=LogInputInterfaceData  DataStoreElements=LogInputInterfaceData.AI_1_Log.log_transPumpTempSens  IndexOptions=Index vector (dialog)  Indices=1  OutputSizes=1
  Data Store Write3 : DataStoreWrite  DataStoreName=InputInterfaceData  DataStoreElements=InputInterfaceData.AI.filterClogSens  IndexOptions=Index vector (dialog)  Indices=1  OutputSizes=1
  Data Store Write30 : DataStoreWrite  DataStoreName=LogInputInterfaceData  DataStoreElements=LogInputInterfaceData.AI_2_Log.log_hydMotTempSens  IndexOptions=Index vector (dialog)  Indices=1  OutputSizes=1
  Data Store Write4 : DataStoreWrite  DataStoreName=UDSStruct  DataStoreElements=UDSStruct.pin_transPumpTempSens  IndexOptions=Index vector (dialog)  Indices=1  OutputSizes=1
  FilterClogSens : TTlibrary/ADC/adcGetValue  adc_channel=IO_ADC_04  types=IO_ADC_RESISTIVE  range=IO_ADC_NO_RANGE  pupd=IO_ADC_NO_PULL  sensor_supply=IO_PIN_NONE  safety_conf=off  adc_val_lower=4  adc_val_upper=4  redundant_channel=IO_ADC_08  io_error=on  sample_time=-1
      settings: SourceProductName=TT control 500 series
  Function Caller19 : FunctionCaller  FunctionPrototype=finalValue = convAIVoltageData(rawValue,errorSts)  InputArgumentSpecifications=<Enter example>  OutputArgumentSpecifications=<Enter example>
  Function Caller26 : FunctionCaller  FunctionPrototype=finalValue = convAIResistanceData(rawValue,errorSts)  InputArgumentSpecifications=<Enter example>  OutputArgumentSpecifications=<Enter example>
  Function Caller6 : FunctionCaller  FunctionPrototype=finalValue = convAIVoltageData(rawValue,errorSts)  InputArgumentSpecifications=<Enter example>  OutputArgumentSpecifications=<Enter example>
  HydromotorTempSens : TTlibrary/ADC/adcGetValue  adc_channel=IO_ADC_22  types=IO_ADC_RATIOMETRIC  range=IO_ADC_RANGE_5V  pupd=IO_ADC_NO_PULL  sensor_supply=IO_SENSOR_SUPPLY_0  safety_conf=off  adc_val_lower=4  adc_val_upper=4  redundant_channel=IO_ADC_08  io_error=on  sample_time=-1
      settings: SourceProductName=TT control 500 series
  Terminator12 : Terminator
  Terminator23 : Terminator
  Terminator3 : Terminator
  TransPumpTempSens : TTlibrary/ADC/adcGetValue  adc_channel=IO_ADC_21  types=IO_ADC_RATIOMETRIC  range=IO_ADC_RANGE_5V  pupd=IO_ADC_NO_PULL  sensor_supply=IO_SENSOR_SUPPLY_0  safety_conf=off  adc_val_lower=4  adc_val_upper=4  redundant_channel=IO_ADC_08  io_error=on  sample_time=-1
      settings: SourceProductName=TT control 500 series
  wires:
  Function Caller26/1 -> Data Store Write26/1, Data Store Write3/1
  FilterClogSens/1 -> Function Caller26/1  "adc_105_value"
  FilterClogSens/3 -> Data Store Write1/1, Function Caller26/2  "adc_105_error"
  FilterClogSens/2 -> Terminator3/1  "adc_105_update"
  HydromotorTempSens/1 -> Function Caller6/1  "adc_114_value"
  Function Caller6/1 -> Data Store Write30/1, Data Store Write12/1
  HydromotorTempSens/2 -> Terminator12/1  "adc_114_update"
  HydromotorTempSens/3 -> Data Store Write2/1, Function Caller6/2  "adc_114_error"
  TransPumpTempSens/2 -> Terminator23/1  "adc_137_update"
  TransPumpTempSens/3 -> Data Store Write4/1, Function Caller19/2  "adc_137_error"
  TransPumpTempSens/1 -> Function Caller19/1  "adc_137_value"
  Function Caller19/1 -> Data Store Write28/1, Data Store Write23/1
